simulink model "AEBDecisionLogic"  (R2022b)
settings: Solver=FixedStepAuto  StartTime=0.0  StopTime=inf  FixedStep=0.05  RelTol=1e-3
undefined symbols (not defined in the file): trackingParams, Ts
settings Model: Creator=The MathWorks, Inc.  LastModifiedBy=The MathWorks, Inc.
settings SolverCC: AlgebraicLoopSolver=TrustRegion  MinimalZcImpactIntegration=on  MaxZcPerStep=1
settings DataIOCC: SaveOutput=off  SignalLogging=off  SaveTime=off  ReturnWorkspaceOutputs=off
settings OptimizationCC: DefaultParameterBehavior=Inlined  InlineInvariantSignals=on  PassReuseOutputArgsAs=Individual arguments  ZeroExternalMemoryAtStartup=off  ZeroInternalMemoryAtStartup=off  OptimizeBlockOrder=speed  EfficientTunableParamExpr=on
settings DebuggingCC: ParameterTunabilityLossMsg=error  UnconnectedInputMsg=warning  UnconnectedOutputMsg=warning  UnconnectedLineMsg=warning  SFMachineParentedDataDiag=warning  ArithmeticOperatorsInVariantConditions=warning
settings HardwareCC: ProdLongLongMode=on
settings ModelReferenceCC: EnableRefExpFcnMdlSchedulingChecks=on  PropagateVarSize=Only when enabling
settings SFSimCC: SimUseLocalCustomCode=off  MATLABDynamicMemAlloc=off  CustomCodeUndefinedFunction=UseInterfaceOnly  SimTargetLang=C++
settings RTWCC: Description=Embedded Coder  SystemTargetFile=ert.tlc  TemplateMakefile=ert_default_tmf  GenerateReport=on  RTWUseLocalCustomCode=off  BuildConfiguration=Faster Runs  IncludeHyperlinkInReport=on  LaunchReport=on  TargetLang=C++  GenerateTraceInfo=on  GenerateTraceReport=on  GenerateTraceReportSl=on  GenerateTraceReportSf=on  GenerateTraceReportEml=on  GenerateCodeMetricsReport=on  DLArmComputeVersion=19.05
settings CodeAppCC: ForceParamTrailComments=on  IgnoreCustomStorageClasses=off  MaxIdLength=63  OperatorAnnotations=on  SimulinkDataObjDesc=on  SFDataObjDesc=on  CustomSymbolStrFcn=$N$M$F  InsertBlockDesc=on
settings ERTTargetCC: TargetLangStandard=C++03 (ISO)  GenerateSampleERTMain=on  CombineSignalStateStructs=on  SuppressErrorStatus=on  CodeInterfacePackaging=C++ class  InlinedParameterPlacement=NonHierarchical  RootIOFormat=Structure reference  RTWCAPISignals=on  ERTCustomFileTemplate=example_file_process.tlc

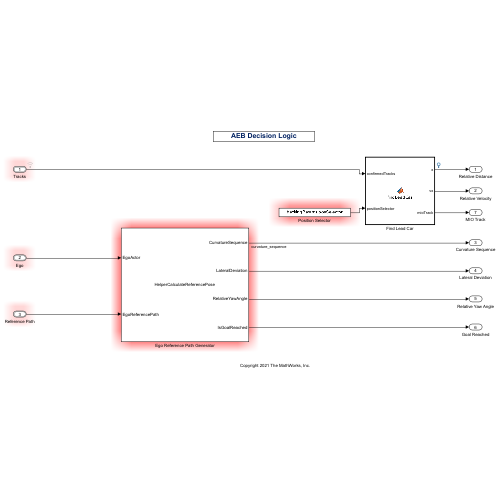
[thumbnail: Simulink's stored preview of the top-level diagram]
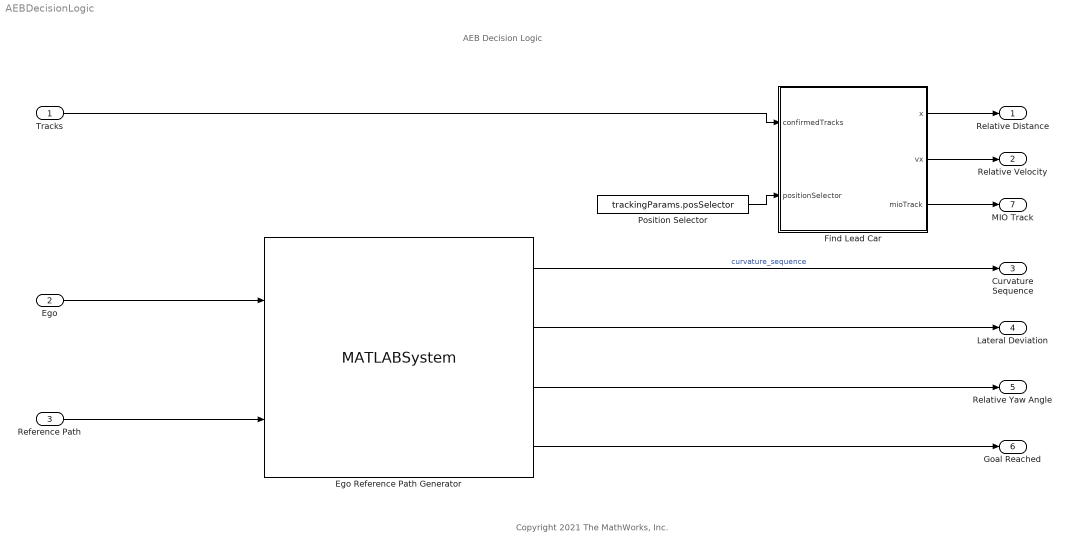
== system AEBDecisionLogic ==
  note: Copyright 2021 The MathWorks, Inc.
  note: AEB Decision Logic
  Tracks : Inport  OutDataTypeStr=Bus: BusMultiObjectTracker1  SampleTime=[Ts, 0]  BusOutputAsStruct=on
  Ego : Inport  Port=2  OutDataTypeStr=Bus: BusVehiclePose
  Reference Path : Inport  Port=3  OutDataTypeStr=Bus: BusEgoRefPath
  Ego Reference Path Generator : MATLABSystem  System=HelperCalculateReferencePose  PredictionHorizon=predictionHorizon  DistanceFromCGToRear=lr  SimulateUsing=Interpreted execution
      mask Type: HelperCalculateReferencePose
      mask Display:
      | disp('HelperCalculateReferencePose');
      | port_label('input',1,'EgoActor');
      | port_label('input',2,'EgoReferencePath');
      | port_label('output',1,'CurvatureSequence');
      | port_label('output',2,'LateralDeviation');
      | port_label('output',3,'RelativeYawAngle');
      | port_label('output',4,'IsGoalReached');
  Find Lead Car : MATLAB Function  TreatAsAtomicUnit=on
  Position Selector : Constant  Value=trackingParams.posSelector
  Relative Distance : Outport
  Relative Velocity : Outport  Port=2
  Curvature Sequence : Outport  Port=3
  Lateral Deviation : Outport  Port=4
  Relative Yaw Angle : Outport  Port=5
  Goal Reached : Outport  Port=6
  MIO Track : Outport  Port=7
  wires:
  Reference Path/1 -> Ego Reference Path Generator/2
  Ego/1 -> Ego Reference Path Generator/1
  Ego Reference Path Generator/2 -> Lateral Deviation/1
  Tracks/1 -> Find Lead Car/1(confirmedTracks)
  Ego Reference Path Generator/4 -> Goal Reached/1
  Find Lead Car/1(x) -> Relative Distance/1
  Ego Reference Path Generator/1 -> Curvature Sequence/1  "curvature_sequence"
  Find Lead Car/2(vx) -> Relative Velocity/1
  Ego Reference Path Generator/3 -> Relative Yaw Angle/1
  Find Lead Car/3(mioTrack) -> MIO Track/1
  Position Selector/1 -> Find Lead Car/2(positionSelector)

== matlab function AEBDecisionLogic/Find Lead Car ==
  data: confirmedTracks input Bus: BusMultiObjectTracker1; x output size=[1 1]; vx output size=[1 1]; mioTrack output; positionSelector input
function [x,vx,mioTrack] = findLeadCar(confirmedTracks, positionSelector)
% This function finds the lead car: a car in front of the ego car that
% satisfies all the criteria below:
% * Within the ego car's lane.
% * In front of the ego car.
% * Closest to the ego car.

% Important notes:
% 1. If you change state definition, change the following:
%       State = [x;vx;y;vy;z;vz] (3D constant velocity)
numStates = 6;

% 2. The lane is defined using a parabolic model, where y=ax^2+bx+c. a is
%    equal to half the road curvature, b=0, and c is the offset of the lane
%    boundaries relative to the ego car. Overall lane width is assumed to
%    be 3.6m, typical highway lane width.
laneWidth = 3.6;

% 3. The ego car is assumed to be traveling in the middle of its lane, with
%    1.8m on each side of it. So, c=+1.8m for the left lane boundary and
%    -1.8m for the right lane boundary.
halfLaneWidth = laneWidth/2;

% Initialize outputs and parameters
maxX = cast(1000, 'like', confirmedTracks.Tracks(1).State);  % Far enough forward so that no track is expected to exceed this distance
trackID = 0;



for i = 1:confirmedTracks.NumTracks
    position = positionSelector * confirmedTracks.Tracks(i).State;
    x = position(1); % Longitudinal position of the track relative to ego
    y = position(2); % Lateral position of the track relative to ego
    
    if x < maxX && x > 0 % No point checking otherwise
        yleftLane  = polyval([0, 0,  halfLaneWidth],x); % Half a lane to the left
        yrightLane = polyval([0, 0, -halfLaneWidth],x); % Half a lane to the right
        
        % Find a new lead car
        if (yrightLane <= y) && (y <= yleftLane)
            maxX = x;
            trackID = i;
        end
    end
end

if trackID>0
    mioState = confirmedTracks.Tracks(trackID).State;
else
    mioState = zeros(numStates,1,'like',confirmedTracks.Tracks(1).State);
    mioState(1) = 500;
    mioState(2) = 0.01;
end

% Output:
x = mioState(1);    % Longitudinal position of the lead car
vx = mioState(2);   % Longitudinal velocity of the lead car
mioTrack = trackID; % Index of the most important track
